simulink model "fuzzy_switch"  (R2024b)
settings: Solver=VariableStepAuto  StartTime=0.0  StopTime=9  RelTol=1e-3
libraries: fuzblock x1
settings Model: Creator=19065  LastModifiedBy=19065

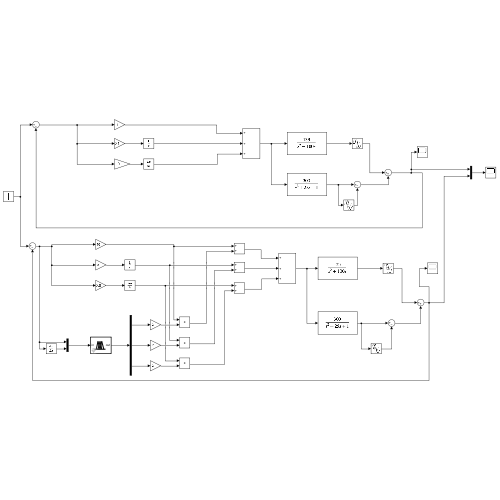
[thumbnail: Simulink's stored preview of the top-level diagram]
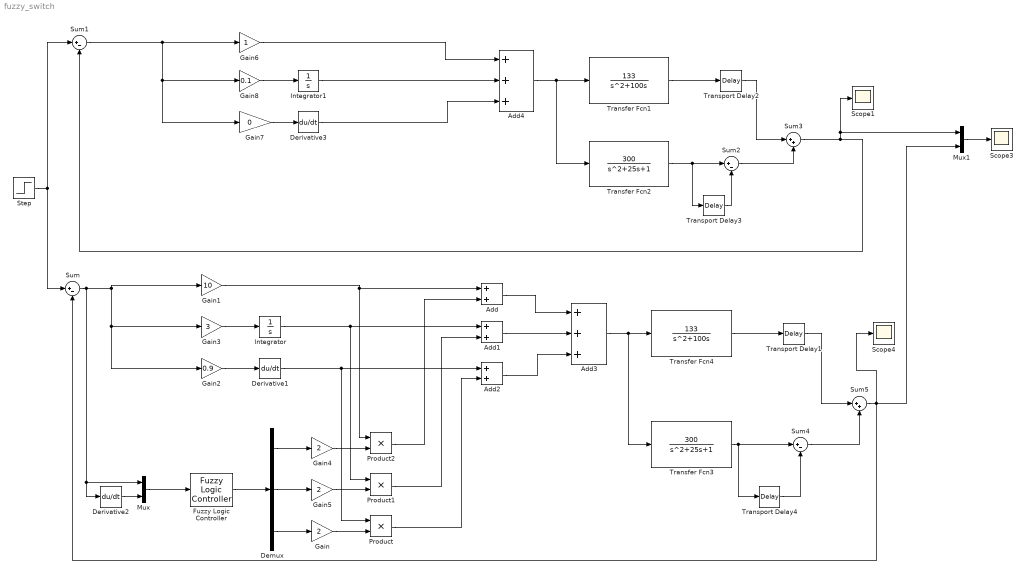
== system fuzzy_switch ==
  Add : Sum
  Add1 : Sum
  Add2 : Sum
  Add3 : Sum  Inputs=+++
  Add4 : Sum  Inputs=+++
  Demux : Demux  Outputs=3
  Derivative1 : Derivative
  Derivative2 : Derivative
  Derivative3 : Derivative
  Fuzzy Logic Controller : fuzblock/Fuzzy Logic  Controller  FIS=fuzzy2  OutputSampleNumber=101  DataType=double  FuzzifiedInputs=off  RuleFiringStrengths=off  RuleOutputs=off  AggregatedOutputs=off  SimulateUsing=Interpreted execution  OutOfRangeInputValueMessage=warning  NoRuleFiredMessage=warning  EmptyOutputFuzzySetMessage=warning
  Gain : Gain  Gain=2
  Gain1 : Gain  Gain=10
  Gain2 : Gain  Gain=0.9
  Gain3 : Gain  Gain=3
  Gain4 : Gain  Gain=2
  Gain5 : Gain  Gain=2
  Gain6 : Gain
  Gain7 : Gain  Gain=0
  Gain8 : Gain  Gain=0.1
  Integrator : Integrator
  Integrator1 : Integrator
  Mux : Mux  Inputs=2
  Mux1 : Mux  Inputs=2
  Product : Product
  Product1 : Product
  Product2 : Product
  Scope1 : Scope
  Scope3 : Scope
  Scope4 : Scope
  Step : Step  Time=0  SampleTime=0
  Sum{,1..2,4} (4 alike) : Sum  Inputs=|+-
  Sum3 : Sum  Inputs=|++
  Sum5 : Sum  Inputs=|++
  Transfer Fcn1 : TransferFcn  Numerator=[133]  Denominator=[1 100 0]
  Transfer Fcn2 : TransferFcn  Numerator=[300]  Denominator=[1 25 1]
  Transfer Fcn3 : TransferFcn  Numerator=[300]  Denominator=[1 25 1]
  Transfer Fcn4 : TransferFcn  Numerator=[133]  Denominator=[1 100 0]
  Transport Delay1 : TransportDelay  DelayTime=5
  Transport Delay2 : TransportDelay  DelayTime=5  BufferSize=1024000
  Transport Delay3 : TransportDelay  DelayTime=5  BufferSize=1024000
  Transport Delay4 : TransportDelay  DelayTime=5
  wires:
  Gain1/1 -> Add/1, Product2/1
  Sum5/1 -> Scope4/1, Sum/2, Mux1/2
  Gain7/1 -> Derivative3/1
  Integrator1/1 -> Add4/2
  Transport Delay1/1 -> Sum5/1
  Fuzzy Logic Controller/1 -> Demux/1
  Sum4/1 -> Sum5/2
  Demux/1 -> Gain4/1
  Derivative3/1 -> Add4/3
  Add/1 -> Add3/1
  Gain6/1 -> Add4/1
  Transfer Fcn4/1 -> Transport Delay1/1
  Product/1 -> Add2/2
  Gain8/1 -> Integrator1/1
  Mux/1 -> Fuzzy Logic Controller/1
  Demux/3 -> Gain/1
  Integrator/1 -> Product1/1, Add1/1
  Derivative2/1 -> Mux/2
  Gain4/1 -> Product2/2
  Transfer Fcn3/1 -> Sum4/1, Transport Delay4/1
  Gain2/1 -> Derivative1/1
  Mux1/1 -> Scope3/1
  Transport Delay2/1 -> Sum3/1
  Sum/1 -> Mux/1, Derivative2/1, Gain2/1, Gain3/1, Gain1/1
  Add1/1 -> Add3/2
  Transfer Fcn1/1 -> Transport Delay2/1
  Add4/1 -> Transfer Fcn2/1, Transfer Fcn1/1
  Demux/2 -> Gain5/1
  Transport Delay3/1 -> Sum2/2
  Sum2/1 -> Sum3/2
  Gain5/1 -> Product1/2
  Transport Delay4/1 -> Sum4/2
  Product2/1 -> Add/2
  Step/1 -> Sum/1, Sum1/1
  Gain/1 -> Product/2
  Add2/1 -> Add3/3
  Gain3/1 -> Integrator/1
  Sum3/1 -> Mux1/1, Scope1/1, Sum1/2
  Derivative1/1 -> Product/1, Add2/1
  Add3/1 -> Transfer Fcn3/1, Transfer Fcn4/1
  Sum1/1 -> Gain7/1, Gain8/1, Gain6/1
  Transfer Fcn2/1 -> Transport Delay3/1, Sum2/1
  Product1/1 -> Add1/2
